simulink library "crs"  (Simulink 8.1)
settings: Solver=ode1  StartTime=0.0  StopTime=Inf  FixedStep=0.001  RelTol=1e-3
PostLoadFcn:
  | , if any(exist('dsrtsu_mdlpostloadfcn', 'file') == [2, 3, 6]), try dsrtsu_mdlpostloadfcn('Execute', bdroot); catch fprintf('Error in PostLoadFcn (dsrtsu_mdlpostloadfcn) for model "%s":\n %s\n', bdroot, lasterr); end, end,
undefined symbols (not defined in the file or in its folder): C_TICK_TIME_S, ENUM_ACCSTATE_STANDSTILL, FALSE, KJUD_ACCAutoRefollowTimer_ms, KJUD_ACCThrottleToStart_pct, KJUD_ACCVehReadyTimer_ms, TRUE, ZERO_INT
libraries: hcu_lib x1
settings Model: DSRTSU_INTERNAL_RTI_VER=450  DSRTSU_INTERNAL_RTI_TYPE=rti1401  RTICANMMDATA=struct('GeneralSetupData',struct('modelroot','D:\ELN150201_TAIWAN\trunk\AdasDragon\software\sw_development\arch\app\jud','generalsettings',struct('filesettings',struct('destfolder',struct('Name','RTICANMM_FILES','Check',1),'buildfolder',struct('Name','.','Check',1),'AbsDestfolder',struct('Name','D:\ELN150201_TAIWAN\trunk\AdasDragon\software\sw_development\arch\app\jud\RTICANMM_FILES'),'AbsBuildfolder',struct('Name','D:\ELN150201_TAIWAN\trunk\AdasDragon\software\sw_development\arch\app\jud'))),'options',struct('addpaths',1,'rmpaths',1,'addtrcexclusion',logical(1),'cannavigator',struct('checkmonitoring',0),'show_usrtrc',0,'use_usrtrc',0),'advanced',struct('options',[1 1 1 1 1 1 1 1 1 1 1 1 1 1 1 1 1 1 1 1 1 1 1 1 1 1 1 1 1 1 1 1 1 1 1 1 1 1 1 1 1 1 1 1 1 1 1 1 1 1 1 1 1 1 1 1 1 1 1 1 1 1 1 1 1 1 1 1 1 1 1 1 1 1 1 1 1 1 1 1 1 1 1 1 1 1 1 1 1 1 1 1 1 1 1 1 1 1 1 1]),'MPSetup',{{}},'modelname','crs','block','crs'))  DSRTSU_INTERNAL_RTIFPGA=40  Creator=AT015411  LastModifiedBy=AT015555

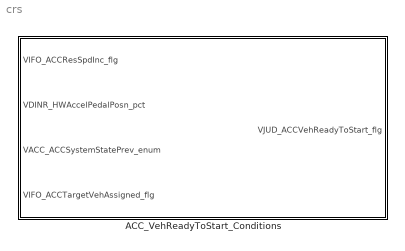
== system crs ==
  ACC_VehReadyToStart_Conditions : Subsystem

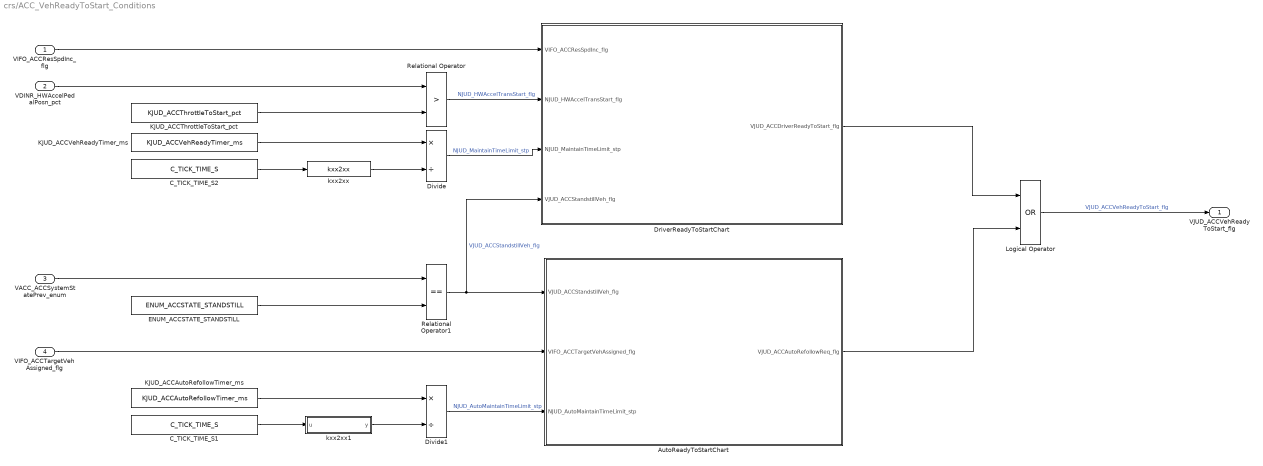
== system crs/ACC_VehReadyToStart_Conditions ==
  VIFO_ACCResSpdInc_flg : Inport
  VDINR_HWAccelPedalPosn_pct : Inport  Port=2
  VACC_ACCSystemStatePrev_enum : Inport  Port=3
  VIFO_ACCTargetVehAssigned_flg : Inport  Port=4
  AutoReadyToStartChart : Stateflow chart  TreatAsAtomicUnit=on
  C_TICK_TIME_S1 : Constant  Value=C_TICK_TIME_S  OutDataTypeStr=single
  C_TICK_TIME_S2 : Constant  Value=C_TICK_TIME_S  OutDataTypeStr=single
  Divide : Product  Inputs=*/
  Divide1 : Product  Inputs=*/
  DriverReadyToStartChart : Stateflow chart  TreatAsAtomicUnit=on
  ENUM_ACCSTATE_STANDSTILL : Constant  Value=ENUM_ACCSTATE_STANDSTILL  OutDataTypeStr=single
  KJUD_ACCAutoRefollowTimer_ms : Constant  Value=KJUD_ACCAutoRefollowTimer_ms  OutDataTypeStr=single
  KJUD_ACCThrottleToStart_pct : Constant  Value=KJUD_ACCThrottleToStart_pct
  KJUD_ACCVehReadyTimer_ms : Constant  Value=KJUD_ACCVehReadyTimer_ms  OutDataTypeStr=single
  Logical Operator : Logic  Operator=OR  AllPortsSameDT=off  OutDataTypeStr=boolean
  Relational Operator : RelationalOperator  Operator=>  OutDataTypeStr=boolean
  Relational Operator1 : RelationalOperator  Operator===  OutDataTypeStr=boolean
  kxx2xx : hcu_lib/kxx2xx
  kxx2xx1 : Subsystem  mask(Conversion){}
      mask help: Multiply by 1000.
      mask Display: disp('kiloxx \rightarrow xx', 'texmode', 'on')
  VJUD_ACCVehReadyToStart_flg : Outport
  wires:
  kxx2xx/1 -> Divide/2
  Divide/1 -> DriverReadyToStartChart/3(NJUD_MaintainTimeLimit_stp)  "NJUD_MaintainTimeLimit_stp"
  C_TICK_TIME_S2/1 -> kxx2xx/1
  KJUD_ACCVehReadyTimer_ms/1 -> Divide/1
  Logical Operator/1 -> VJUD_ACCVehReadyToStart_flg/1  "VJUD_ACCVehReadyToStart_flg"
  VIFO_ACCResSpdInc_flg/1 -> DriverReadyToStartChart/1(VIFO_ACCResSpdInc_flg)
  Relational Operator/1 -> DriverReadyToStartChart/2(NJUD_HWAccelTransStart_flg)  "NJUD_HWAccelTransStart_flg"
  VDINR_HWAccelPedalPosn_pct/1 -> Relational Operator/1
  KJUD_ACCThrottleToStart_pct/1 -> Relational Operator/2
  VACC_ACCSystemStatePrev_enum/1 -> Relational Operator1/1
  ENUM_ACCSTATE_STANDSTILL/1 -> Relational Operator1/2
  kxx2xx1/1(y) -> Divide1/2
  C_TICK_TIME_S1/1 -> kxx2xx1/1(u)
  KJUD_ACCAutoRefollowTimer_ms/1 -> Divide1/1
  Relational Operator1/1 -> DriverReadyToStartChart/4(VJUD_ACCStandstillVeh_flg), AutoReadyToStartChart/1(VJUD_ACCStandstillVeh_flg)  "VJUD_ACCStandstillVeh_flg"
  VIFO_ACCTargetVehAssigned_flg/1 -> AutoReadyToStartChart/2(VIFO_ACCTargetVehAssigned_flg)
  Divide1/1 -> AutoReadyToStartChart/3(NJUD_AutoMaintainTimeLimit_stp)  "NJUD_AutoMaintainTimeLimit_stp"
  AutoReadyToStartChart/1(VJUD_ACCAutoRefollowReq_flg) -> Logical Operator/2
  DriverReadyToStartChart/1(VJUD_ACCDriverReadyToStart_flg) -> Logical Operator/1

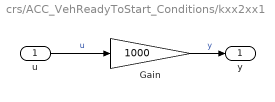
== system crs/ACC_VehReadyToStart_Conditions/kxx2xx1 ==
  u : Inport
  Gain : Gain  Gain=1000
  y : Outport
  wires:
  u/1 -> Gain/1  "u"
  Gain/1 -> y/1  "y"

== stateflow chart ACC_VehReadyToStart_Conditions/DriverReadyToStartChart ==
  state ON
    en:
    VJUD_ACCDriverReadyToStart_flg = TRUE;
  state MAINTAIN
    en:
    NJUD_MaintainTimeLocal_stp = ZERO_INT;
    du:
    NJUD_MaintainTimeLocal_stp = NJUD_MaintainTimeLocal_stp+1;
  state OFF
    en:
    VJUD_ACCDriverReadyToStart_flg = FALSE;
  (default) -> OFF
  (junction 15) -> OFF : [NJUD_MaintainTimeLocal_stp>=NJUD_MaintainTimeLimit_stp]
  MAINTAIN -> (junction 15) [order 2]
  OFF -> (junction 16)
  ON -> MAINTAIN : [VIFO_ACCResSpdInc_flg==FALSE...
      | && NJUD_HWAccelTransStart_flg==FALSE]
  (junction 16) -> ON : [(VIFO_ACCResSpdInc_flg==TRUE...
      | || NJUD_HWAccelTransStart_flg==TRUE)...
      | && VJUD_ACCStandstillVeh_flg == TRUE]
  MAINTAIN -> ON [order 1] : [VIFO_ACCResSpdInc_flg==TRUE...
      | || NJUD_HWAccelTransStart_flg==TRUE]
  data: VIFO_ACCResSpdInc_flg input boolean; VJUD_ACCDriverReadyToStart_flg output boolean; NJUD_HWAccelTransStart_flg input boolean; NJUD_MaintainTimeLimit_stp input single; TRUE parameter boolean; FALSE parameter boolean; NJUD_MaintainTimeLocal_stp local single; ZERO_INT parameter double; VJUD_ACCStandstillVeh_flg input double

== stateflow chart ACC_VehReadyToStart_Conditions/AutoReadyToStartChart ==
  state RUNNING
    en:
    VJUD_ACCAutoRefollowReq_flg = FALSE;
  state STOPPED
    en:
    VJUD_ACCAutoRefollowReq_flg = TRUE;
    NJUD_AutoMaintainTimeLocal_stp=ZERO_INT;
    du:
    NJUD_AutoMaintainTimeLocal_stp=NJUD_AutoMaintainTimeLocal_stp+1;
  state LONG_STOPPED
    en:
    VJUD_ACCAutoRefollowReq_flg = FALSE;
  (default) -> RUNNING
  RUNNING -> STOPPED : [VJUD_ACCStandstillVeh_flg==TRUE...
      | && VIFO_ACCTargetVehAssigned_flg==TRUE]
  STOPPED -> LONG_STOPPED [order 2] : [NJUD_AutoMaintainTimeLocal_stp>=NJUD_AutoMaintainTimeLimit_stp]
  STOPPED -> RUNNING [order 1] : [VIFO_ACCTargetVehAssigned_flg==FALSE...
      | || VJUD_ACCStandstillVeh_flg==FALSE]
  LONG_STOPPED -> RUNNING : [VIFO_ACCTargetVehAssigned_flg==FALSE...
      | || VJUD_ACCStandstillVeh_flg==FALSE]
  data: VJUD_ACCAutoRefollowReq_flg output boolean; TRUE parameter boolean; FALSE parameter boolean; VJUD_ACCStandstillVeh_flg input boolean; VIFO_ACCTargetVehAssigned_flg input double; NJUD_AutoMaintainTimeLocal_stp local double; NJUD_AutoMaintainTimeLimit_stp input double; ZERO_INT parameter double
